simulink model "RM3_w_DD"  (R2014b)
settings: Solver=ode4  StartTime=0  StopTime=300  FixedStep=0.001  RelTol=1e-3
undefined symbols (not defined in the file or in its folder): body, constraint, pto
libraries: WECSim_Lib x5, PTOSim_Lib x1
settings Model: Creator=mlawson  LastModifiedBy=rso
settings SolverCC: AlgebraicLoopSolver=LineSearch
settings DataIOCC: LimitDataPoints=off  SaveOutput=off  SaveTime=off
settings DebuggingCC: UnderspecifiedInitializationDetection=Classic  MergeDetectMultiDrivingBlocksExec=none  StateNameClashWarn=warning
settings ExplorerConfigSet: InternalSimMechanicsExplorerSettings="<ExplorerConfiguration><canonicalview>default</canonicalview><TilePanel><TileInfo><Tiles Columns=\"1\" Count=\"1\" Rows=\"1\"><Column Left=\"2\" Weight=\"1\"/><Column Left=\"1335\"/><Row Top=\"2\" Weight=\"1\"/><Row Top=\"911\"/><Tile Height=\"1\" Width=\"1\" X=\"0\" Y=\"0\"/></Tiles></TileInfo><SceneInfo><SceneViewer><BGColor><R>0.60000002384185791</R><G>0.60000002384185791</G><B>0.60000002384185791</B></BGColor><Camera><Position><X>365.37645888990272</X><Y>-369.82486814446582</Y><Z>359.64809521743916</Z></Position><Center><X>-6.7351450971904585</X><Y>2.2867358426280204</Y><Z>-12.463508769654169</Z></Center><Up><X>-0.40824829046386307</X><Y>0.40824829046386307</Y><Z>0.81649658092772615</Z></Up><Left>-57.820127362122818</Left><Right>57.820127362122818</Right><Bottom>-38.308817187253304</Bottom><Top>38.308817187253304</Top></Camera></SceneViewer></SceneInfo></TilePanel></ExplorerConfiguration>"

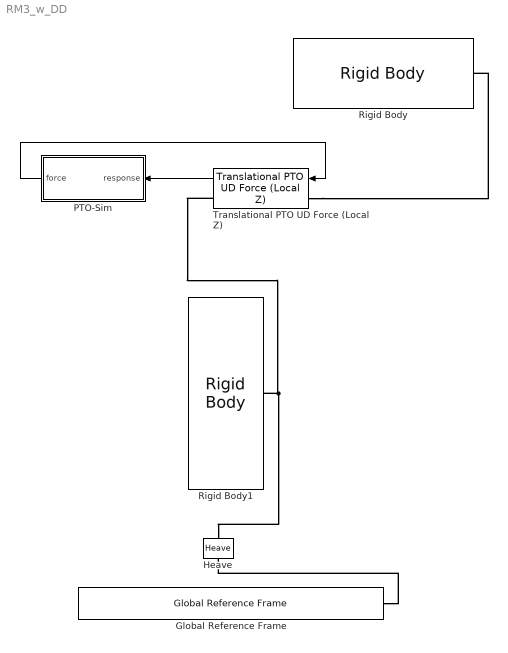
== system RM3_w_DD ==
  Global Reference Frame : WECSim_Lib/Frames/Global Reference Frame  waves=waves  simu=simu
  Heave : WECSim_Lib/Constraints/Heave  constraint=constraint(1)
      settings: AttributesFormatString=%<constraint>
  PTO-Sim : Subsystem  mask{Parameter=0}
  Rigid Body : WECSim_Lib/Body Elements/Rigid Body  body=body(1)
      settings: AttributesFormatString=%<body>
  Rigid Body1 : WECSim_Lib/Body Elements/Rigid Body  body=body(2)
      settings: AttributesFormatString=%<body>
  Translational PTO UD Force (Local Z) : WECSim_Lib/PTOs/Translational PTO UD Force  (Local Z)  pto=pto(1)
      settings: AttributesFormatString=%<pto>
  wires:
  Translational PTO UD Force (Local Z)/1 -> PTO-Sim/1(response)
  PTO-Sim/1(force) -> Translational PTO UD Force (Local Z)/1
  connections:
  Global Reference Frame/RConn1 -- Heave/LConn1
  Rigid Body1/RConn1 -- Translational PTO UD Force (Local Z)/RConn1 -- Heave/RConn1
  Translational PTO UD Force (Local Z)/LConn1 -- Rigid Body/RConn1

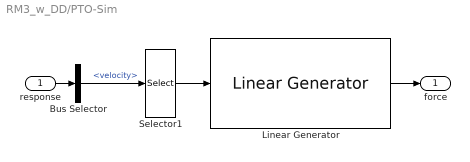
== system RM3_w_DD/PTO-Sim ==
  response : Inport
  Bus Selector : BusSelector  OutputSignals=velocity
  Linear Generator : PTOSim_Lib/ Generator/Linear Generator  ptosim=ptosim.linearGenerator
  Selector1 : Selector  InputPortWidth=6  Indices=3
  force : Outport
  wires:
  Linear Generator/1 -> force/1
  response/1 -> Bus Selector/1
  Bus Selector/1 -> Selector1/1  "<velocity>"
  Selector1/1 -> Linear Generator/1
